simulink model "Kalman_LV_Test1"  (R2025a)
settings: Solver=VariableStepAuto  StartTime=0.0  StopTime=10  FixedStep=0.001  RelTol=1e-3
libraries: slpidlib x3
settings Model: Creator=benjaminlevin  LastModifiedBy=benjaminlevin

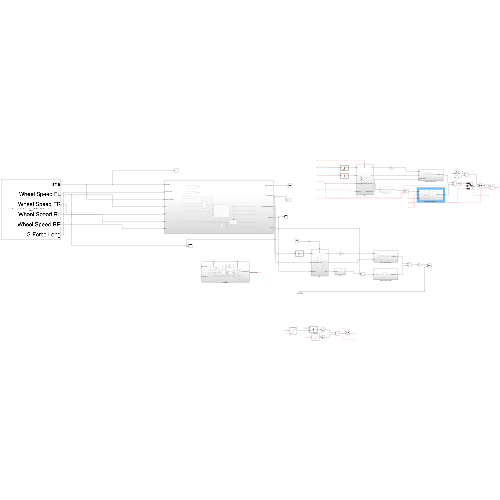
[thumbnail: Simulink's stored preview of the top-level diagram]
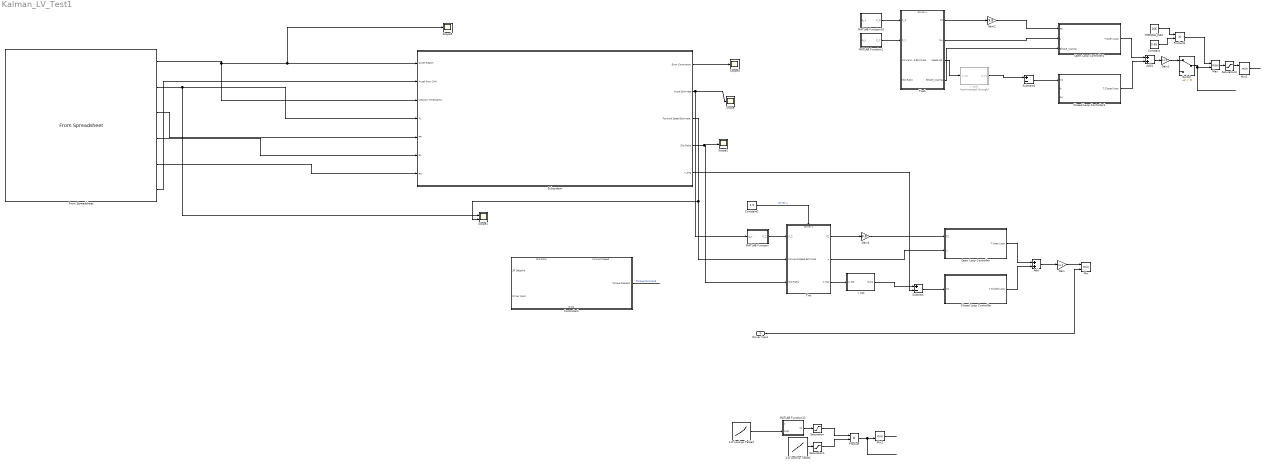
== system Kalman_LV_Test1 ==
  Driver Input : Inport
  1-D Lookup Table1 : Lookup_n-D  NumberOfTableDimensions=1  BreakpointsForDimension1=[1;10]  Table=[0;166]  ExtrapMethod=Clip  InternalRulePriority=Speed  RndMeth=Simplest
  1-D Lookup Table2 : Lookup_n-D  NumberOfTableDimensions=1  BreakpointsForDimension1=[1;10]  Table=[0.03;0.21]  ExtrapMethod=Clip  InternalRulePriority=Speed  RndMeth=Simplest
  Add : Sum
  Add1 : Sum
  Closed Loop Controller : Subsystem
  Closed Loop Controller1 : Subsystem
  Constant : Constant  Value=0.65
  Constant1 : Constant  Value=1.5
  Controller1 : Subsystem
      settings: PortSchema="{\"entries\":[{\"content\":{\"sides\":[{\"content\":{\"connectorIds\":[\"In1\",\"In2\"]},\"type\":\"ConnectorPlacement.EquallySpacedRectSide\",\"uuid\":\"c0b03cac-8500-440b-9ad3-70bdbcbe41b3\"},{\"content\":{\"connectorIds\":[\"Out1\"],\"side\":\"RIGHT\"},\"type\":\"ConnectorPlacement.EquallySpacedRectSide\",\"uuid\":\"4e59df84-775e-4047-ac34-66ccc124485b\"},{\"content\":{\"connectorIds\":[\"In3\",\"In4\"],\"side\":\"TOP\"},\"type\":\"ConnectorPlacement.EquallySpacedRectSide\",\"uuid\":\"12bec3c0-59ce-461e-8d83-22bbad6940ac\"},{\"content\":{\"connectorIds\":[\"Out2\"],\"side\":\"BOTTOM\"},\"type\":\"ConnectorPlacement.EquallySpacedRectSide\",\"uuid\":\"5f001fec-b6eb-40c7-946e-6a0b01bf2b52\"}]},\"type\":\"ConnectorPlacement.EquallySpacedConnector\",\"uuid\":\"2aa18406-4382-4098-896d-4e093aea1de1\"}],\"packageUris\":[\"http://schema.mathworks.com/mf0/Connector/R2020b\"],\"version\":\"1.0\"}"
  From Spreadsheet : FromSpreadsheet  FileName=/Users/benjaminlevin/Downloads/Formula SAE/KalmanMatTestSuyash.xlsx  TreatFirstColumnAs=Data  SampleTime=0.002
  Gain : Gain  Gain=1/4.9
  Gain1 : Gain  Gain=1/4.9
  Gain2 : Gain  Gain=9.8
  Gain3 : Gain  Gain=9.8
  MATLAB Function : MATLAB Function  TreatAsAtomicUnit=on
  MATLAB Function1 : MATLAB Function  TreatAsAtomicUnit=on
  MATLAB Function10 : MATLAB Function  TreatAsAtomicUnit=on
  MATLAB Function11 : MATLAB Function  TreatAsAtomicUnit=on
  Max : MinMax  Function=max  Inputs=2
  Min : MinMax  Inputs=2
  Min1 : MinMax  Inputs=2
  Min2 : MinMax  Inputs=2
  Open Loop Controller : Subsystem
  Open Loop Controller1 : Subsystem
  Product : Product
  Product1 : Product
  Saturation : Saturate  UpperLimit=1  LowerLimit=.1
  Saturation1 : Saturate  UpperLimit=166  LowerLimit=0
  Saturation2 : Saturate  UpperLimit=166  LowerLimit=0
  Scope{,2,4..5} (4 alike) : Scope
      Scope settings: ActiveDisplayYMinimum=-0.4138  ActiveDisplayYMaximum=3.5361
      Scope2 settings: ActiveDisplayYMinimum=-0.10736  ActiveDisplayYMaximum=0.13295  DataLoggingVariableName=ScopeData2
      Scope4 settings: ActiveDisplayYMinimum=-1910.81188  ActiveDisplayYMaximum=17197.30688
      Scope5 settings: ActiveDisplayYMinimum=-1.25  ActiveDisplayYMaximum=11.25
  Scope1 : Scope  NumInputPorts=2
      settings: ActiveDisplayYMinimum=-4.95  ActiveDisplayYMaximum=44.55
  Subsystem : Subsystem
  Subtract : Sum  Inputs=+-
  Subtract1 : Sum  Inputs=+-
  Switch : Switch  Criteria=u2 > Threshold  SaturateOnIntegerOverflow=off  InputSameDT=off
  TORQUE_MAX : Constant  Value=166
  Tire : Subsystem
      settings: PortSchema="{\"entries\":[{\"content\":{\"sides\":[{\"content\":{\"connectorIds\":[\"In1\",\"In2\",\"In3\"]},\"type\":\"ConnectorPlacement.EquallySpacedRectSide\",\"uuid\":\"4156dcb8-571a-4ee4-a7f1-7560a1681aa7\"},{\"content\":{\"connectorIds\":[\"Out1\",\"Out2\",\"Out3\"],\"side\":\"RIGHT\"},\"type\":\"ConnectorPlacement.EquallySpacedRectSide\",\"uuid\":\"73638d28-b906-4671-b83f-ad6b48e8d393\"},{\"content\":{\"connectorIds\":[\"In4\"],\"side\":\"TOP\"},\"type\":\"ConnectorPlacement.EquallySpacedRectSide\",\"uuid\":\"2e0ca522-3e79-4dd0-9128-59b05a2bd3de\"}]},\"type\":\"ConnectorPlacement.EquallySpacedConnector\",\"uuid\":\"62676716-b41d-4cd9-a12c-b09e0afde3e3\"}],\"packageUris\":[\"http://schema.mathworks.com/mf0/Connector/R2020b\"],\"version\":\"1.0\"}"
  Tire1 : Subsystem
      settings: PortSchema="{\"entries\":[{\"content\":{\"sides\":[{\"content\":{\"connectorIds\":[\"In1\",\"In2\",\"In3\",\"In4\"]},\"type\":\"ConnectorPlacement.EquallySpacedRectSide\",\"uuid\":\"4156dcb8-571a-4ee4-a7f1-7560a1681aa7\"},{\"content\":{\"connectorIds\":[\"Out1\",\"Out2\",\"Out3\",\"Out4\"],\"side\":\"RIGHT\"},\"type\":\"ConnectorPlacement.EquallySpacedRectSide\",\"uuid\":\"73638d28-b906-4671-b83f-ad6b48e8d393\"},{\"content\":{\"connectorIds\":[\"In5\"],\"side\":\"TOP\"},\"type\":\"ConnectorPlacement.EquallySpacedRectSide\",\"uuid\":\"2e0ca522-3e79-4dd0-9128-59b05a2bd3de\"}]},\"type\":\"ConnectorPlacement.EquallySpacedConnector\",\"uuid\":\"62676716-b41d-4cd9-a12c-b09e0afde3e3\"}],\"packageUris\":[\"http://schema.mathworks.com/mf0/Connector/R2020b\"],\"version\":\"1.0\"}"
  v opt : Subsystem
  v opt1 : Subsystem  Commented=through
  wires:
  Subsystem/3(Forward Speed Estimate) -> Tire/2(Forward Speed Estimate), Scope1/2
  Subsystem/1(Error Covariance) -> Scope4/1
  Subsystem/4(Slip Ratio) -> Tire/3(Slip Ratio), Scope2/1
  Subsystem/2(Accel Estimate) -> Scope/1, MATLAB Function/1(a_x)
  From Spreadsheet/2 -> Subsystem/4(FL), Scope1/1
  From Spreadsheet/5 -> Subsystem/7(RR)
  Controller1/1(Torque Request) -> ?  "Torque Command"
  Open Loop Controller/1(T Open Loop) -> Add/1
  Closed Loop Controller/1(T Closed Loop) -> Add/2
  Add/1 -> Gain/1
  Driver Input/1 -> Min/2
  Subsystem/5(v_avg) -> Subtract/2
  MATLAB Function/1(F_Z) -> Tire/1(F_Z)
  Gain/1 -> Min/1
  Tire/3(w opt) -> v opt/1(w opt)
  v opt/1(Out1) -> Subtract/1
  Subtract/1 -> Closed Loop Controller/1(In1)
  Tire/1(FZ) -> Gain3/1
  Tire/2(u) -> Open Loop Controller/2(u)
  Constant1/1 -> Tire/4(Driver u)  "Driver u"
  From Spreadsheet/6 -> Subsystem/2(Accel from CAN)
  From Spreadsheet/1 -> Scope5/1, Subsystem/1(Accel Report), Subsystem/3(Velocity Timestamp)
  From Spreadsheet/3 -> Subsystem/5(FR)
  From Spreadsheet/4 -> Subsystem/6(RL)
  ? -> 1-D Lookup Table2/1
  ? -> MATLAB Function11/1(k)
  Min1/1 -> ?
  Saturation/1 -> Product/1
  Saturation1/1 -> Product/2
  1-D Lookup Table1/1 -> Saturation1/1
  ? -> Min1/1
  ? -> 1-D Lookup Table1/1
  Product/1 -> Min1/2
  MATLAB Function11/1(TF) -> Saturation/1
  1-D Lookup Table2/1 -> MATLAB Function11/2(kopt)
  Tire1/4(Ellipse_scaling) -> Open Loop Controller1/3(Ellipse_scaling)
  ? -> MATLAB Function1/1(a_y)
  MATLAB Function1/1(F_Y) -> Tire1/2(F_Y)
  Product1/1 -> Max/1
  Constant/1 -> Product1/2
  TORQUE_MAX/1 -> Product1/1
  Max/1 -> Saturation2/1
  ? -> Closed Loop Controller1/2(Ki)
  Min2/1 -> ?
  ? -> Min2/2, Switch/3
  Switch/1 -> Max/2
  ? -> Switch/2, Tire1/3(Forward Speed Estimate)
  Gain2/1 -> Open Loop Controller1/1(FZ)
  Saturation2/1 -> Min2/1
  ? -> Closed Loop Controller1/3(Kp)
  ? -> Tire1/4(Slip Ratio)
  ? -> Subtract1/2
  ? -> Tire1/5(Driver u)
  Tire1/1(FZ) -> Gain2/1
  Add1/1 -> Gain1/1
  Subtract1/1 -> Closed Loop Controller1/1(In1)
  Tire1/3(speed opt) -> v opt1/1(w opt)
  v opt1/1(Out1) -> Subtract1/1
  Closed Loop Controller1/1(T Closed Loop) -> Add1/2
  Open Loop Controller1/1(T Open Loop) -> Add1/1
  MATLAB Function10/1(F_Z) -> Tire1/1(F_Z)
  ? -> MATLAB Function10/1(a_x)
  Tire1/2(mu) -> Open Loop Controller1/2(u)
  Gain1/1 -> Switch/1
  Gain3/1 -> Open Loop Controller/1(FZ)

== system Kalman_LV_Test1/Closed Loop Controller ==
  In1 : Inport
  PID Controller : slpidlib/PID Controller  Controller=PID  Form=Parallel  TimeDomain=Discrete-time  UseExternalTs=off  SampleTime=-1  IntegratorMethod=Forward Euler  FilterMethod=Forward Euler  ControllerParametersSource=internal  P=100  I=10  UseKiTs=off  D=0  UseExternalDerivativeSource=off  N=100  UseFilter=on  TunerSelectOption=Transfer Function Based (PID Tuner App)  InitialConditionSource=internal  InitialConditionForIntegrator=0  InitialConditionForFilter=0  DifferentiatorICPrevScaledInput=0  ExternalReset=none  TrackingMode=off  Kt=1  LimitOutput=on  SatLimitsSource=internal  UpperSaturationLimit=inf  LowerSaturationLimit=-inf  LinearizeAsGain=on  AntiWindupMode=clamping  Kb=1  LimitIntegrator=off  UpperIntegratorSaturationLimit=inf  LowerIntegratorSaturationLimit=-inf  POutMin=[]  POutMax=[]  IOutMin=[]  IOutMax=[]  DOutMin=[]  DOutMax=[]  NOutMin=[]  NOutMax=[]  SumOutMin=[]  SumOutMax=[]  SaturationOutMin=[]  SaturationOutMax=[]  PParamMin=[]  PParamMax=[]  IParamMin=[]  IParamMax=[]  DParamMin=[]  DParamMax=[]  NParamMin=[]  NParamMax=[]  KbParamMin=[]  KbParamMax=[]  KtParamMin=[]  KtParamMax=[]  KbOutMin=[]  KbOutMax=[]  KtOutMin=[]  KtOutMax=[]  IntegratorOutMin=[]  IntegratorOutMax=[]  FilterOutMin=[]  FilterOutMax=[]  SumI1OutMin=[]  SumI1OutMax=[]  SumI2OutMin=[]  SumI2OutMax=[]  SumI3OutMin=[]  SumI3OutMax=[]  SumI4OutMin=[]  SumI4OutMax=[]  SumDOutMin=[]  SumDOutMax=[]  DifferentiatorOutMin=[]  DifferentiatorOutMax=[]  FilterDiffOutCoefMin=[]  FilterDiffOutCoefMax=[]  ReciprocalOutMin=[]  ReciprocalOutMax=[]  SumDenOutMin=[]  SumDenOutMax=[]  SumNumOutMin=[]  SumNumOutMax=[]  DivideOutMin=[]  DivideOutMax=[]  UdiffTsProdOutMin=[]  UdiffTsProdOutMax=[]  NTsProdOutMin=[]  NTsProdOutMax=[]  UintegralTsProdOutMin=[]  UintegralTsProdOutMax=[]  UngainTsProdOutMin=[]  UngainTsProdOutMax=[]  ClampingZeroOutDataTypeStr=Inherit: Inherit via back propagation  ClampingZeroOutMin=[]  ClampingZeroOutMax=[]  FilterDenConstantOutDataTypeStr=Inherit: Inherit via back propagation  FilterDenConstantOutMin=[]  FilterDenConstantOutMax=[]  PCopyOutDataTypeStr=Inherit: Inherit via back propagation  PCopyOutMin=[]  PCopyOutMax=[]  NCopyOutDataTypeStr=Inherit: Inherit via back propagation  NCopyOutMin=[]  NCopyOutMax=[]  IntegratorContinuousStateAttributes=''  IntegratorStateMustResolveToSignalObject=off  IntegratorRTWStateStorageClass=Auto  FilterContinuousStateAttributes=''  FilterStateMustResolveToSignalObject=off  FilterRTWStateStorageClass=Auto  ParallelPVariant=InternalParameters  IdealPVariant=Disabled  IVariant=InternalParameters  DVariant=InternalParameters  IntegratorVariant=Discrete  SatVariant=Enabled  AWVariant=DiscClampingParallel  PCopyVariant=Disabled  TRVariant=Disabled  FdbkBlocksVariant=Forward  IdealPFdbkVariant=Disabled  SatFdbkVariant=Disabled  DerivativeFilterVariant=ForwardEulerFilter  NVariant=InternalParameters  NCopyVariant=Disabled  FilterICVariant=InternalICsFilter  IntegratorICVariant=InternalICs  ExternalResetVariant=Disabled  TRSumVariant=Passthrough  SumFdbkVariant=Disabled  SumVariant=Sum_PID  TsampFilterVariant=InternalTs  TsampNgainVariant=Passthrough  TsampIntegralVariant=Disabled_SignalSpec  ExternalSaturationOutDataTypeStr=Inherit: Same as second input  DerivativeSourceVariant=ErrorSignal  PreIntVariant=InternalPreInt
  T Closed Loop : Outport
  wires:
  In1/1 -> PID Controller/1
  PID Controller/1 -> T Closed Loop/1

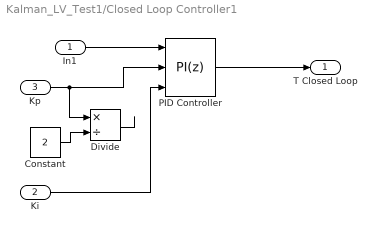
== system Kalman_LV_Test1/Closed Loop Controller1 ==
  In1 : Inport
  Ki : Inport  Port=2
  Kp : Inport  Port=3
  Constant : Constant  Value=2
  Divide : Product  Inputs=*/
  PID Controller : slpidlib/PID Controller  Controller=PI  Form=Parallel  TimeDomain=Discrete-time  UseExternalTs=off  SampleTime=-1  IntegratorMethod=Forward Euler  FilterMethod=Forward Euler  ControllerParametersSource=external  P=100  I=10  UseKiTs=off  D=0  UseExternalDerivativeSource=off  N=100  UseFilter=on  TunerSelectOption=Transfer Function Based (PID Tuner App)  InitialConditionSource=internal  InitialConditionForIntegrator=0  InitialConditionForFilter=0  DifferentiatorICPrevScaledInput=0  ExternalReset=none  TrackingMode=off  Kt=1  LimitOutput=on  SatLimitsSource=internal  UpperSaturationLimit=166  LowerSaturationLimit=0  LinearizeAsGain=on  AntiWindupMode=clamping  Kb=1  LimitIntegrator=on  UpperIntegratorSaturationLimit=166  LowerIntegratorSaturationLimit=0  POutMin=[]  POutMax=[]  IOutMin=[]  IOutMax=[]  DOutMin=[]  DOutMax=[]  NOutMin=[]  NOutMax=[]  SumOutMin=[]  SumOutMax=[]  SaturationOutMin=[]  SaturationOutMax=[]  PParamMin=[]  PParamMax=[]  IParamMin=[]  IParamMax=[]  DParamMin=[]  DParamMax=[]  NParamMin=[]  NParamMax=[]  KbParamMin=[]  KbParamMax=[]  KtParamMin=[]  KtParamMax=[]  KbOutMin=[]  KbOutMax=[]  KtOutMin=[]  KtOutMax=[]  IntegratorOutMin=[]  IntegratorOutMax=[]  FilterOutMin=[]  FilterOutMax=[]  SumI1OutMin=[]  SumI1OutMax=[]  SumI2OutMin=[]  SumI2OutMax=[]  SumI3OutMin=[]  SumI3OutMax=[]  SumI4OutMin=[]  SumI4OutMax=[]  SumDOutMin=[]  SumDOutMax=[]  DifferentiatorOutMin=[]  DifferentiatorOutMax=[]  FilterDiffOutCoefMin=[]  FilterDiffOutCoefMax=[]  ReciprocalOutMin=[]  ReciprocalOutMax=[]  SumDenOutMin=[]  SumDenOutMax=[]  SumNumOutMin=[]  SumNumOutMax=[]  DivideOutMin=[]  DivideOutMax=[]  UdiffTsProdOutMin=[]  UdiffTsProdOutMax=[]  NTsProdOutMin=[]  NTsProdOutMax=[]  UintegralTsProdOutMin=[]  UintegralTsProdOutMax=[]  UngainTsProdOutMin=[]  UngainTsProdOutMax=[]  ClampingZeroOutDataTypeStr=Inherit: Inherit via back propagation  ClampingZeroOutMin=[]  ClampingZeroOutMax=[]  FilterDenConstantOutDataTypeStr=Inherit: Inherit via back propagation  FilterDenConstantOutMin=[]  FilterDenConstantOutMax=[]  PCopyOutDataTypeStr=Inherit: Inherit via back propagation  PCopyOutMin=[]  PCopyOutMax=[]  NCopyOutDataTypeStr=Inherit: Inherit via back propagation  NCopyOutMin=[]  NCopyOutMax=[]  IntegratorContinuousStateAttributes=''  IntegratorStateMustResolveToSignalObject=off  IntegratorRTWStateStorageClass=Auto  FilterContinuousStateAttributes=''  FilterStateMustResolveToSignalObject=off  FilterRTWStateStorageClass=Auto  ParallelPVariant=ExternalParameters  IdealPVariant=Disabled  IVariant=ExternalParameters  DVariant=Disabled  IntegratorVariant=Discrete  SatVariant=Enabled  AWVariant=DiscClampingParallel  PCopyVariant=Disabled  TRVariant=Disabled  FdbkBlocksVariant=Forward  IdealPFdbkVariant=Disabled  SatFdbkVariant=Disabled  DerivativeFilterVariant=Disabled  NVariant=Disabled  NCopyVariant=Disabled_SignalSpec  FilterICVariant=Disabled  IntegratorICVariant=InternalICs  ExternalResetVariant=Disabled  TRSumVariant=Passthrough  SumFdbkVariant=Disabled  SumVariant=Sum_PI  TsampFilterVariant=InternalTs  TsampNgainVariant=Passthrough  TsampIntegralVariant=Disabled_SignalSpec  ExternalSaturationOutDataTypeStr=Inherit: Same as second input  DerivativeSourceVariant=Disabled  PreIntVariant=InternalPreInt
  T Closed Loop : Outport
  wires:
  In1/1 -> PID Controller/1
  PID Controller/1 -> T Closed Loop/1
  Kp/1 -> Divide/1, PID Controller/2
  Divide/1 -> ?
  Constant/1 -> Divide/2
  Ki/1 -> PID Controller/3

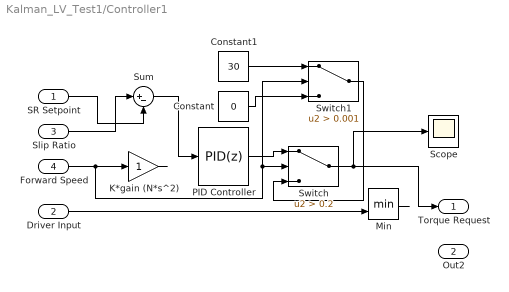
== system Kalman_LV_Test1/Controller1 ==
  SR Setpoint : Inport
  Driver Input : Inport  Port=2
  Slip Ratio : Inport  Port=3
  Forward Speed : Inport  Port=4
  Constant : Constant  Value=0
  Constant1 : Constant  Value=30
  K*gain (N*s^2) : Gain
  Min : MinMax  Inputs=2
  PID Controller : slpidlib/PID Controller  Controller=PID  Form=Parallel  TimeDomain=Discrete-time  UseExternalTs=off  SampleTime=-1  IntegratorMethod=Forward Euler  FilterMethod=Forward Euler  ControllerParametersSource=internal  P=100  I=10  UseKiTs=off  D=0  UseExternalDerivativeSource=off  N=100  UseFilter=on  TunerSelectOption=Transfer Function Based (PID Tuner App)  InitialConditionSource=internal  InitialConditionForIntegrator=0  InitialConditionForFilter=0  DifferentiatorICPrevScaledInput=0  ExternalReset=none  TrackingMode=off  Kt=1  LimitOutput=on  SatLimitsSource=internal  UpperSaturationLimit=inf  LowerSaturationLimit=-inf  LinearizeAsGain=on  AntiWindupMode=clamping  Kb=1  LimitIntegrator=off  UpperIntegratorSaturationLimit=inf  LowerIntegratorSaturationLimit=-inf  POutMin=[]  POutMax=[]  IOutMin=[]  IOutMax=[]  DOutMin=[]  DOutMax=[]  NOutMin=[]  NOutMax=[]  SumOutMin=[]  SumOutMax=[]  SaturationOutMin=[]  SaturationOutMax=[]  PParamMin=[]  PParamMax=[]  IParamMin=[]  IParamMax=[]  DParamMin=[]  DParamMax=[]  NParamMin=[]  NParamMax=[]  KbParamMin=[]  KbParamMax=[]  KtParamMin=[]  KtParamMax=[]  KbOutMin=[]  KbOutMax=[]  KtOutMin=[]  KtOutMax=[]  IntegratorOutMin=[]  IntegratorOutMax=[]  FilterOutMin=[]  FilterOutMax=[]  SumI1OutMin=[]  SumI1OutMax=[]  SumI2OutMin=[]  SumI2OutMax=[]  SumI3OutMin=[]  SumI3OutMax=[]  SumI4OutMin=[]  SumI4OutMax=[]  SumDOutMin=[]  SumDOutMax=[]  DifferentiatorOutMin=[]  DifferentiatorOutMax=[]  FilterDiffOutCoefMin=[]  FilterDiffOutCoefMax=[]  ReciprocalOutMin=[]  ReciprocalOutMax=[]  SumDenOutMin=[]  SumDenOutMax=[]  SumNumOutMin=[]  SumNumOutMax=[]  DivideOutMin=[]  DivideOutMax=[]  UdiffTsProdOutMin=[]  UdiffTsProdOutMax=[]  NTsProdOutMin=[]  NTsProdOutMax=[]  UintegralTsProdOutMin=[]  UintegralTsProdOutMax=[]  UngainTsProdOutMin=[]  UngainTsProdOutMax=[]  ClampingZeroOutDataTypeStr=Inherit: Inherit via back propagation  ClampingZeroOutMin=[]  ClampingZeroOutMax=[]  FilterDenConstantOutDataTypeStr=Inherit: Inherit via back propagation  FilterDenConstantOutMin=[]  FilterDenConstantOutMax=[]  PCopyOutDataTypeStr=Inherit: Inherit via back propagation  PCopyOutMin=[]  PCopyOutMax=[]  NCopyOutDataTypeStr=Inherit: Inherit via back propagation  NCopyOutMin=[]  NCopyOutMax=[]  IntegratorContinuousStateAttributes=''  IntegratorStateMustResolveToSignalObject=off  IntegratorRTWStateStorageClass=Auto  FilterContinuousStateAttributes=''  FilterStateMustResolveToSignalObject=off  FilterRTWStateStorageClass=Auto  ParallelPVariant=InternalParameters  IdealPVariant=Disabled  IVariant=InternalParameters  DVariant=InternalParameters  IntegratorVariant=Discrete  SatVariant=Enabled  AWVariant=DiscClampingParallel  PCopyVariant=Disabled  TRVariant=Disabled  FdbkBlocksVariant=Forward  IdealPFdbkVariant=Disabled  SatFdbkVariant=Disabled  DerivativeFilterVariant=ForwardEulerFilter  NVariant=InternalParameters  NCopyVariant=Disabled  FilterICVariant=InternalICsFilter  IntegratorICVariant=InternalICs  ExternalResetVariant=Disabled  TRSumVariant=Passthrough  SumFdbkVariant=Disabled  SumVariant=Sum_PID  TsampFilterVariant=InternalTs  TsampNgainVariant=Passthrough  TsampIntegralVariant=Disabled_SignalSpec  ExternalSaturationOutDataTypeStr=Inherit: Same as second input  DerivativeSourceVariant=ErrorSignal  PreIntVariant=InternalPreInt
  Scope : Scope
      settings: ActiveDisplayYMinimum=-679.77779  ActiveDisplayYMaximum=443.59482  DataLoggingVariableName=ScopeData2
  Sum : Sum  Inputs=|+-
  Switch : Switch  Criteria=u2 > Threshold  Threshold=0.2  SaturateOnIntegerOverflow=off  InputSameDT=off
  Switch1 : Switch  Criteria=u2 > Threshold  Threshold=0.001  SaturateOnIntegerOverflow=off  InputSameDT=off
  Torque Request : Outport
  Out2 : Outport  Port=2
  wires:
  Slip Ratio/1 -> Sum/1
  Sum/1 -> PID Controller/1
  PID Controller/1 -> Switch/1
  Min/1 -> ?
  SR Setpoint/1 -> Sum/2
  Driver Input/1 -> Min/2
  K*gain (N*s^2)/1 -> ?
  Constant1/1 -> Switch1/1
  Forward Speed/1 -> Switch1/2, Switch/2, K*gain (N*s^2)/1
  Switch/1 -> Torque Request/1, Scope/1
  Constant/1 -> Switch1/3
  Switch1/1 -> Switch/3

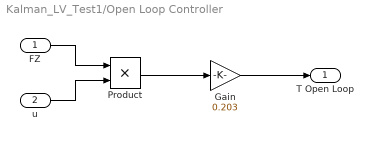
== system Kalman_LV_Test1/Open Loop Controller ==
  FZ : Inport
  u : Inport  Port=2
  Gain : Gain  Gain=0.203
  Product : Product
  T Open Loop : Outport
  wires:
  FZ/1 -> Product/1
  u/1 -> Product/2
  Product/1 -> Gain/1
  Gain/1 -> T Open Loop/1

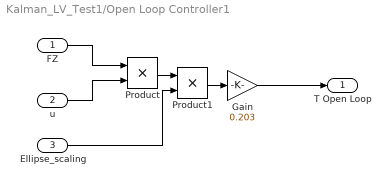
== system Kalman_LV_Test1/Open Loop Controller1 ==
  FZ : Inport
  u : Inport  Port=2
  Ellipse_scaling : Inport  Port=3
  Gain : Gain  Gain=0.203
  Product : Product
  Product1 : Product
  T Open Loop : Outport
  wires:
  FZ/1 -> Product/1
  u/1 -> Product/2
  Product/1 -> Product1/1
  Gain/1 -> T Open Loop/1
  Product1/1 -> Gain/1
  Ellipse_scaling/1 -> Product1/2

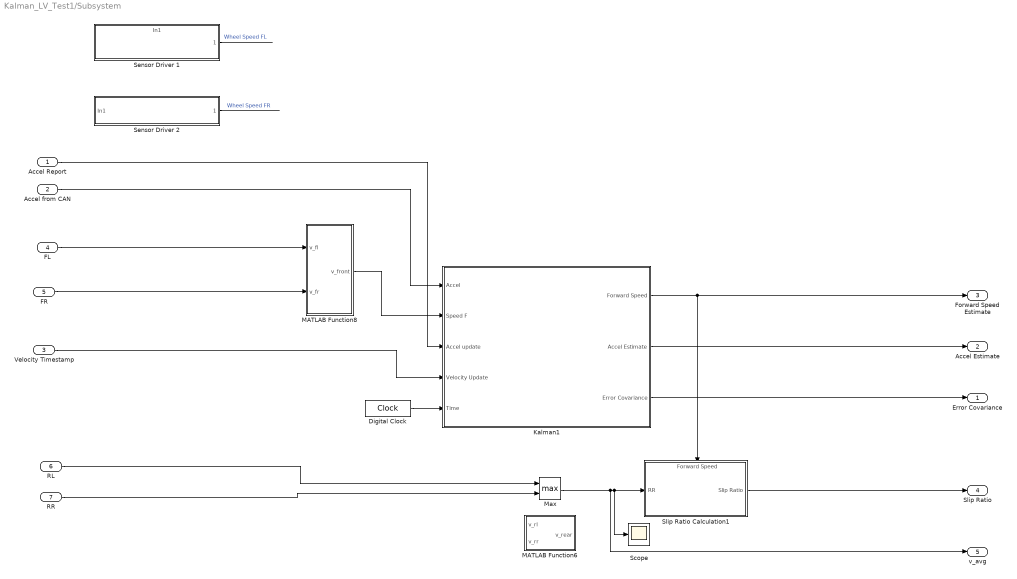
== system Kalman_LV_Test1/Subsystem ==
  Accel Report : Inport
  Accel from CAN : Inport  Port=2
  Velocity Timestamp : Inport  Port=3
  FL : Inport  Port=4
  FR : Inport  Port=5
  RL : Inport  Port=6
  RR : Inport  Port=7
  Digital Clock : DigitalClock  SampleTime=.001
  Kalman1 : Subsystem
  MATLAB Function6 : MATLAB Function  TreatAsAtomicUnit=on
  MATLAB Function8 : MATLAB Function  TreatAsAtomicUnit=on
  Max : MinMax  Function=max  Inputs=2
  Scope : Scope
      settings: ActiveDisplayYMinimum=-5.0375  ActiveDisplayYMaximum=45.3375  DataLoggingVariableName=ScopeData3
  Sensor Driver 1 : Subsystem
      settings: PortSchema="{\"entries\":[{\"content\":{\"sides\":[{\"content\":{},\"type\":\"ConnectorPlacement.EquallySpacedRectSide\",\"uuid\":\"2033c98e-71df-4793-b993-d07749140985\"},{\"content\":{\"connectorIds\":[\"Out1\"],\"side\":\"RIGHT\"},\"type\":\"ConnectorPlacement.EquallySpacedRectSide\",\"uuid\":\"23e09764-9572-407a-9fbd-4abc4e8d3f9a\"},{\"content\":{\"connectorIds\":[\"In1\"],\"side\":\"TOP\"},\"type\":\"ConnectorPlacement.EquallySpacedRectSide\",\"uuid\":\"03519e6f-6b3c-4169-a95a-6bf0e96eeae3\"}]},\"type\":\"ConnectorPlacement.EquallySpacedConnector\",\"uuid\":\"fd32df56-721a-4574-a5c8-784eec41bb92\"}],\"packageUris\":[\"http://schema.mathworks.com/mf0/Connector/R2020b\"],\"version\":\"1.0\"}"
  Sensor Driver 2 : Subsystem
  Slip Ratio Calculation1 : Subsystem
      settings: PortSchema="{\"entries\":[{\"content\":{\"sides\":[{\"content\":{\"connectorIds\":[\"In1\"]},\"type\":\"ConnectorPlacement.EquallySpacedRectSide\",\"uuid\":\"061c82cd-7e9c-4a72-b965-43235230dad9\"},{\"content\":{\"connectorIds\":[\"Out1\"],\"side\":\"RIGHT\"},\"type\":\"ConnectorPlacement.EquallySpacedRectSide\",\"uuid\":\"899eaa50-1c30-4f77-9d66-a8daefd9f1e3\"},{\"content\":{\"connectorIds\":[\"In2\"],\"side\":\"TOP\"},\"type\":\"ConnectorPlacement.EquallySpacedRectSide\",\"uuid\":\"89c07a25-5c36-4b16-a58e-7fbb1fd4b8e3\"}]},\"type\":\"ConnectorPlacement.EquallySpacedConnector\",\"uuid\":\"4f00da10-bd17-48bb-8760-fc873e4c20ca\"}],\"packageUris\":[\"http://schema.mathworks.com/mf0/Connector/R2020b\"],\"version\":\"1.0\"}"
  Error Covariance : Outport
  Accel Estimate : Outport  Port=2
  Forward Speed Estimate : Outport  Port=3
  Slip Ratio : Outport  Port=4
  v_avg : Outport  Port=5
  wires:
  Kalman1/1(Forward Speed) -> Slip Ratio Calculation1/2(Forward Speed), Forward Speed Estimate/1
  Slip Ratio Calculation1/1(Slip Ratio) -> Slip Ratio/1
  FR/1 -> MATLAB Function8/2(v_fr)
  Sensor Driver 2/1(" ") -> ?  "Wheel Speed FR"
  RL/1 -> Max/1
  Sensor Driver 1/1(" ") -> ?  "Wheel Speed FL"
  MATLAB Function8/1(v_front) -> Kalman1/2(Speed F)
  FL/1 -> MATLAB Function8/1(v_fl)
  Accel from CAN/1 -> Kalman1/1(Accel)
  RR/1 -> Max/2
  Digital Clock/1 -> Kalman1/5(Time)
  Kalman1/2(Accel Estimate) -> Accel Estimate/1
  Kalman1/3(Error Covariance) -> Error Covariance/1
  Velocity Timestamp/1 -> Kalman1/4(Velocity Update)
  Accel Report/1 -> Kalman1/3(Accel update)
  Max/1 -> v_avg/1, Scope/1, Slip Ratio Calculation1/1(RR)

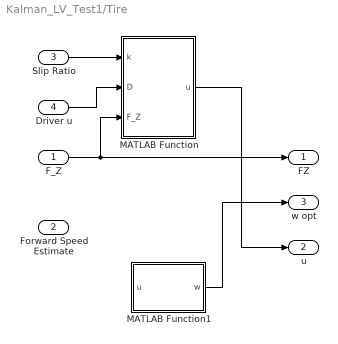
== system Kalman_LV_Test1/Tire ==
  F_Z : Inport
  Forward Speed Estimate : Inport  Port=2
  Slip Ratio : Inport  Port=3
  Driver u : Inport  Port=4
  MATLAB Function : MATLAB Function  TreatAsAtomicUnit=on
  MATLAB Function1 : MATLAB Function  TreatAsAtomicUnit=on
  FZ : Outport
  u : Outport  Port=2
  w opt : Outport  Port=3
  wires:
  F_Z/1 -> MATLAB Function/3(F_Z), FZ/1
  Driver u/1 -> MATLAB Function/2(D)
  Slip Ratio/1 -> MATLAB Function/1(k)
  MATLAB Function/1(u) -> u/1
  MATLAB Function1/1(w) -> w opt/1

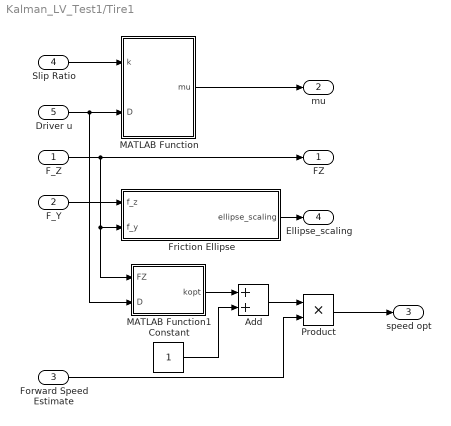
== system Kalman_LV_Test1/Tire1 ==
  F_Z : Inport
  F_Y : Inport  Port=2
  Forward Speed Estimate : Inport  Port=3
  Slip Ratio : Inport  Port=4
  Driver u : Inport  Port=5
  Add : Sum
  Constant : Constant
  Friction Ellipse : MATLAB Function  TreatAsAtomicUnit=on
  MATLAB Function : MATLAB Function  TreatAsAtomicUnit=on
  MATLAB Function1 : MATLAB Function  TreatAsAtomicUnit=on
  Product : Product
  FZ : Outport
  mu : Outport  Port=2
  speed opt : Outport  Port=3
  Ellipse_scaling : Outport  Port=4
  wires:
  F_Z/1 -> FZ/1, Friction Ellipse/2(f_y), MATLAB Function1/1(FZ)
  Driver u/1 -> MATLAB Function/2(D), MATLAB Function1/2(D)
  Slip Ratio/1 -> MATLAB Function/1(k)
  MATLAB Function/1(mu) -> mu/1
  Constant/1 -> Add/2
  MATLAB Function1/1(kopt) -> Add/1
  Add/1 -> Product/1
  Forward Speed Estimate/1 -> Product/2
  Product/1 -> speed opt/1
  F_Y/1 -> Friction Ellipse/1(f_z)
  Friction Ellipse/1(ellipse_scaling) -> Ellipse_scaling/1

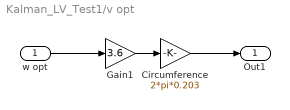
== system Kalman_LV_Test1/v opt ==
  w opt : Inport
  Circumference : Gain  Gain=2*pi*0.203
  Gain1 : Gain  Gain=3.6
  Out1 : Outport
  wires:
  Circumference/1 -> Out1/1
  w opt/1 -> Gain1/1
  Gain1/1 -> Circumference/1

== system Kalman_LV_Test1/v opt1 ==
  w opt : Inport
  Circumference : Gain  Gain=2*pi*0.203
  Gain1 : Gain  Gain=3.6
  Out1 : Outport
  wires:
  Circumference/1 -> Out1/1
  w opt/1 -> Gain1/1
  Gain1/1 -> Circumference/1

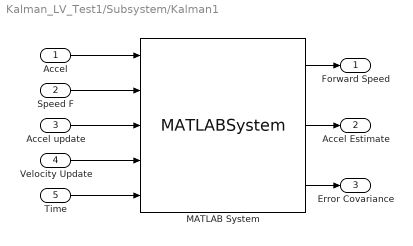
== system Kalman_LV_Test1/Subsystem/Kalman1 ==
  Accel : Inport
  Speed F : Inport  Port=2
  Accel update : Inport  Port=3
  Velocity Update : Inport  Port=4
  Time : Inport  Port=5
  MATLAB System : MATLABSystem  System=Kalman_Filter_Mod  qgain=1  SimulateUsing=Code generation
  Forward Speed : Outport
  Accel Estimate : Outport  Port=2
  Error Covariance : Outport  Port=3
  wires:
  Speed F/1 -> MATLAB System/2
  Accel/1 -> MATLAB System/1
  MATLAB System/1 -> Forward Speed/1
  Accel update/1 -> MATLAB System/3
  Velocity Update/1 -> MATLAB System/4
  Time/1 -> MATLAB System/5
  MATLAB System/2 -> Accel Estimate/1
  MATLAB System/3 -> Error Covariance/1

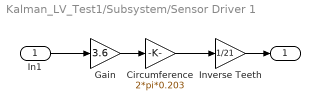
== system Kalman_LV_Test1/Subsystem/Sensor Driver 1 ==
  In1 : Inport
  Circumference : Gain  Gain=2*pi*0.203
  Gain : Gain  Gain=3.6
  Inverse Teeth : Gain  Gain=1/21
  " " : Outport
  wires:
  In1/1 -> Gain/1
  Gain/1 -> Circumference/1
  Circumference/1 -> Inverse Teeth/1
  Inverse Teeth/1 -> " "/1

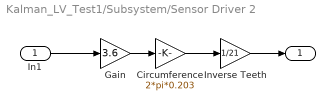
== system Kalman_LV_Test1/Subsystem/Sensor Driver 2 ==
  In1 : Inport
  Circumference : Gain  Gain=2*pi*0.203
  Gain : Gain  Gain=3.6
  Inverse Teeth : Gain  Gain=1/21
  " " : Outport
  wires:
  Circumference/1 -> Inverse Teeth/1
  Inverse Teeth/1 -> " "/1
  In1/1 -> Gain/1
  Gain/1 -> Circumference/1

== system Kalman_LV_Test1/Subsystem/Slip Ratio Calculation1 ==
  RR : Inport
  Forward Speed : Inport  Port=2
  MATLAB Function : MATLAB Function  TreatAsAtomicUnit=on
  Slip Ratio : Outport
  wires:
  Forward Speed/1 -> MATLAB Function/1(fwd_speed)
  RR/1 -> MATLAB Function/2(v_rear)
  MATLAB Function/1(y) -> Slip Ratio/1

== matlab function Kalman_LV_Test1/MATLAB Function ==
  data: a_x input; F_Z output
function F_Z = fcn(a_x)
m = 250+68; %Mass with driver weight
a = 1.530/2; %Distance cg to front axle with load distribution of 0.5
h = 0.249; %Height of CG
l = 1.530; %Length of wheelbase
F_Z = m*(2*a+h*a_x)/(2*l);

== matlab function Kalman_LV_Test1/Tire/MATLAB Function ==
  data: k input; u output; D input; F_Z input
function u = fcn(k,D,F_Z)
B = 1;
E = 1;
C = 1;
F_X = D*sin(C*arctan(B*k-E*(B*k-arctan(B*k))));
u = F_X/F_Z;

== matlab function Kalman_LV_Test1/Tire/MATLAB Function1 ==
  data: u input; w output
function w = fcn(u)
% something blah differential this(B - E*(B - B/(B^2*k^2 + 1)))/((B*k + E*(atan(B*k) - B*k))^2 + 1)
w = u;

== matlab function Kalman_LV_Test1/Subsystem/MATLAB Function6 ==
  data: v_rl input; v_rear output; v_rr input
function v_rear = fcn(v_rl,v_rr)
if(v_rl == 0)
    v_rear = v_rr;
elseif(v_rr == 0)
    v_rear = v_rl;
else
    v_rear= (v_rl+v_rr)/2;
end
end

== matlab function Kalman_LV_Test1/Subsystem/MATLAB Function8 ==
  data: v_fl input; v_front output; v_fr input
function v_front = fcn(v_fl,v_fr)

if(v_fl == 0)
    v_front = v_fr;
elseif(v_fr == 0)
    v_front = v_fl;
else
    v_front= (v_fl+v_fr)/2;
end
end

== matlab function Kalman_LV_Test1/Subsystem/Slip Ratio Calculation1/MATLAB Function ==
  data: fwd_speed input; y output; v_rear input
function y = fcn(fwd_speed,v_rear)

y = (v_rear - fwd_speed)/(max([fwd_speed,0.1]));

== matlab function Kalman_LV_Test1/MATLAB Function1 ==
  data: a_y input; F_Y output
function F_Y = fcn(a_y)
m = 250+68; %Mass with driver weight
a = 1.530/2; %Distance cg to front axle with load distribution of 0.5
h = 0.249; %Height of CG
l = 1.530; %Length of wheelbase
F_Y = (a/l)*m*a_y;

== matlab function Kalman_LV_Test1/MATLAB Function10 ==
  data: a_x input; F_Z output
function F_Z = fcn(a_x)
m = 250+68; %Mass with driver weight
a = 1.530/2; %Distance cg to front axle with load distribution of 0.5
h = 0.249; %Height of CG
l = 1.530; %Length of wheelbase
F_Z = m*(2*a+h*a_x)/(2*l);

== matlab function Kalman_LV_Test1/Tire1/MATLAB Function ==
  data: k input; mu output; D input
function mu = fcn(k,D)
C=1.5926; % [1]
B=11.8721; % [1]
E=0;
mu = D*sin(C*atan(B*k-E*(B*k-atan(B*k))));

== matlab function Kalman_LV_Test1/Tire1/MATLAB Function1 ==
  data: FZ input; D input; kopt output
function kopt = fcn(FZ, D)
% something blah differential this(B - E*(B - B/(B^2*k^2 + 1)))/((B*k + E*(atan(B*k) - B*k))^2 + 1)

B = 7.9557; C = 1.9778; D = 2142.5492; E = 0.3682;

persistent k;
if isempty(k)
    k = 0;
end

if k < 0
    k = 0;
end

T = sin(C*atan(B*k-E*(B*k-atan(B*k))));
dT_dk = (C*cos(C*atan(B*k + E*(atan(B*k) - B*k)))*(B - E*(B - B/(B^2*k^2 + 1))))/((B*k + E*(atan(B*k) - B*k))^2 + 1);

if abs(dT_dk) > 0.05
    k = k + 0.01 * dT_dk;
end


kopt = k;

== matlab function Kalman_LV_Test1/Tire1/Friction Ellipse ==
  data: f_z input; f_y input; ellipse_scaling output
function ellipse_scaling = fcn(f_z, f_y)
u_ymax = 1.36;
ellipse_scaling = sqrt(1-(f_y/(u_ymax*f_z))^2);

== matlab function Kalman_LV_Test1/MATLAB Function11 ==
  data: k input; TF output; kopt input
function TF = fcn(k, kopt)
r=.025;
if (k < kopt-r)
    TF = 1-(kopt-r-k)*0.8;
elseif (k > kopt+r)
    TF = 1-(k-kopt-r)*1.2;
else
    TF = 1;
end
